simulink model "TRAS_closed_loop_"  (R2024b)
settings: Solver=FixedStepAuto  StartTime=0.0  StopTime=stop_time  FixedStep=sampling_time  RelTol=1e-3
values from neighbouring files (symbols this model uses):
  A = 0.0552    [momentsOfInertia.m]
  B = 0.0599    [momentsOfInertia.m]
  C = 0.0084    [momentsOfInertia.m]
  D = (mmr + mms + mm / 3) * lm^2 + (mtr + mts + mt / 3) * lt^2    (= 0.0224143186667)    [momentsOfInertia.m]
  E = mcb * lcb^2 + mb * lb^2 / 3    (= 0.0006225)    [momentsOfInertia.m]    (also in propeller_model.m = 12)
  F = mms * rms^2 + mts * rts^2    (= 0.002355075)    [momentsOfInertia.m]
  Fh_of_u2 = [zeros(1, len - length(Fh_of_u2)), Fh_of_u2] + [zeros(1, len - length(term)), term]    [thrustForcesDependencies.m]
  Fv_of_u1 = [zeros(1, len - length(Fv_of_u1)), Fv_of_u1] + [zeros(1, len - length(term)), term]    [thrustForcesDependencies.m]
  g = 9.81    [TRAS_closed_loop.m]    (also in TRAS_controller.m; TRAS_process.m)
  Jv = D + E + F    (= 0.0253918936667)    [momentsOfInertia.m]
  kd = 2 * zeta * wn + pole    (= 8.88888888889)    [TRAS_closed_loop.m]    (also in TRAS_controller.m = 4)
  kp = wn^2 + 2 * zeta * wn * pole    (= 15.890260631)    [TRAS_closed_loop.m]    (also in TRAS_controller.m = 4)
  L = (mmr + mms + mm / 4) * lm^2 + (mtr + mts + mt / 4) * lt^2 - mcb * lcb^2 - mb / 4 * lb^2    (= 0.021593306)    [momentsOfInertia.m]
  lm = 0.202    [momentsOfInertia.m]
  lt = 0.216    [momentsOfInertia.m]
  sampling_time = 1e-2    (= 0.01)    [TRAS_closed_loop.m]    (also in TRAS_controller.m; TRAS_process.m = 0.001; identification.m)
  x_grid = linspace(-4000, 4000, 1e4)    [TRAS_closed_loop.m]    (also in TRAS_controller.m = linspace(-1, 1, 1e5))
  y_grid_h = polyval(Fh, x_grid)    [TRAS_closed_loop.m]    (also in TRAS_controller.m = polyval(Fh_of_u2, x_grid))
  y_grid_v = polyval(Fv, x_grid)    [TRAS_closed_loop.m]    (also in TRAS_controller.m = polyval(Fv_of_u1, x_grid))
libraries: simulink x2, eeGeneralControl x2
settings Model: Creator=Codrin  LastModifiedBy=Codrin

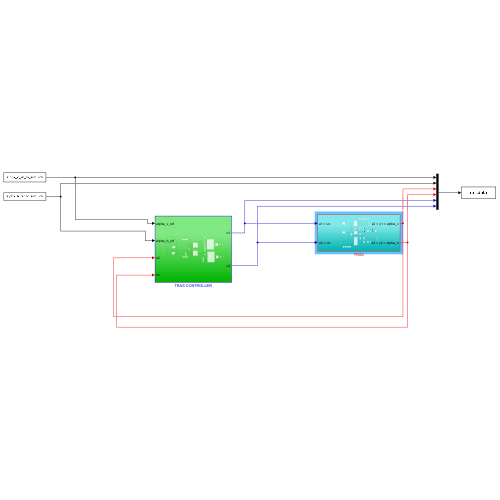
[thumbnail: Simulink's stored preview of the top-level diagram]
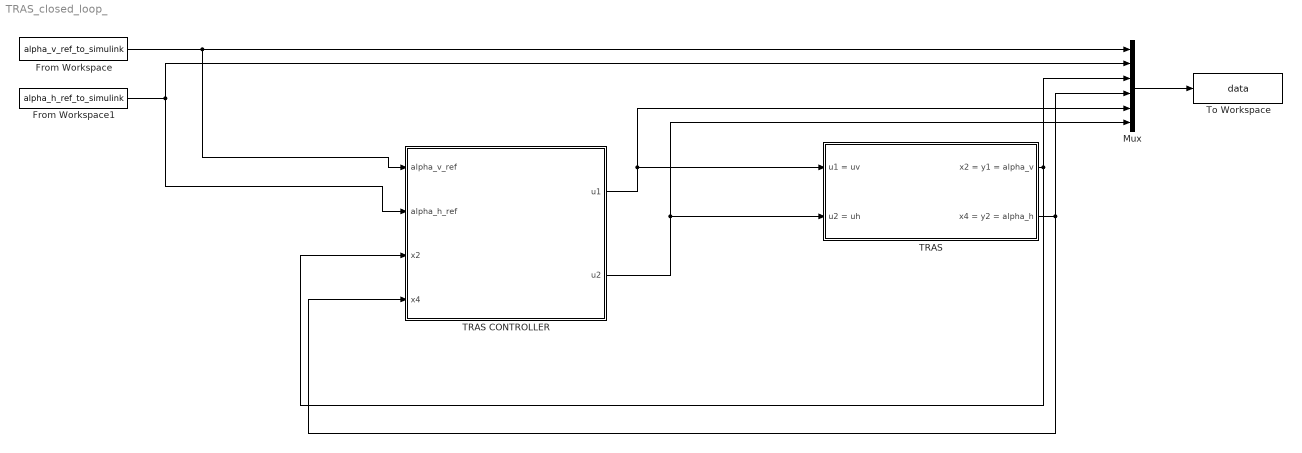
== system TRAS_closed_loop_ ==
  From Workspace : FromWorkspace  VariableName=alpha_v_ref_to_simulink
  From Workspace1 : FromWorkspace  VariableName=alpha_h_ref_to_simulink
  Mux : Mux  Inputs=6
  TRAS : Subsystem
  TRAS CONTROLLER : Subsystem
  To Workspace : ToWorkspace  VariableName=data  SaveFormat=Timeseries  SampleTime=-1
  wires:
  TRAS/2(x4 = y2 = alpha_h) -> TRAS CONTROLLER/4(x4), Mux/4
  Mux/1 -> To Workspace/1
  TRAS/1(x2 = y1 = alpha_v) -> TRAS CONTROLLER/3(x2), Mux/3
  TRAS CONTROLLER/1(u1) -> Mux/5, TRAS/1(u1 = uv)
  TRAS CONTROLLER/2(u2) -> Mux/6, TRAS/2(u2 = uh)
  From Workspace/1 -> TRAS CONTROLLER/1(alpha_v_ref), Mux/1
  From Workspace1/1 -> TRAS CONTROLLER/2(alpha_h_ref), Mux/2

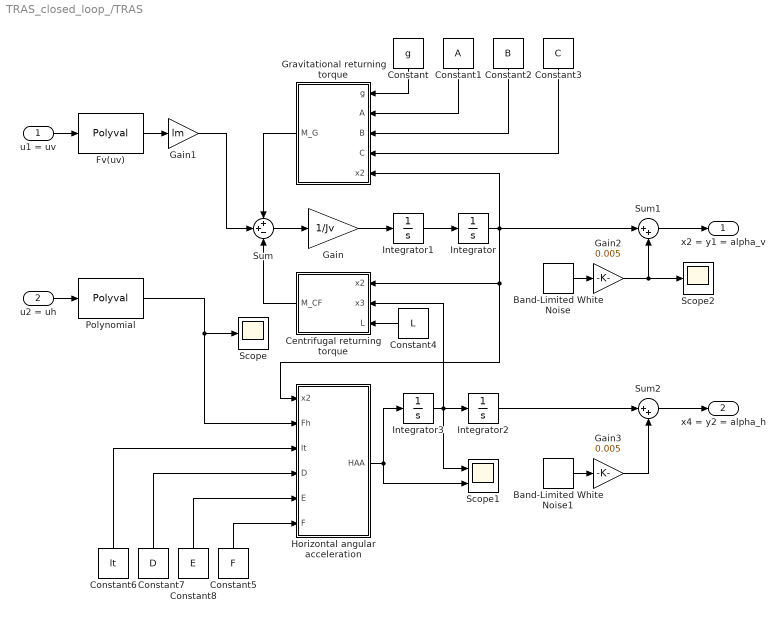
== system TRAS_closed_loop_/TRAS ==
  u1 = uv : Inport
  u2 = uh : Inport  Port=2
  Band-Limited White Noise : simulink/Sources/Band-Limited White Noise  Cov=[0.01]  Ts=sampling_time  seed=[23341]
  Band-Limited White Noise1 : simulink/Sources/Band-Limited White Noise  Cov=[0.01]  Ts=sampling_time  seed=[23341]
  Centrifugal returning torque : MATLAB Function  TreatAsAtomicUnit=on
  Constant : Constant  Value=g
  Constant1 : Constant  Value=A
  Constant2 : Constant  Value=B
  Constant3 : Constant  Value=C
  Constant4 : Constant  Value=L
  Constant5 : Constant  Value=F
  Constant6 : Constant  Value=lt
  Constant7 : Constant  Value=D
  Constant8 : Constant  Value=E
  Fv(uv) : Polyval  Coefs=Fv_of_u1
  Gain : Gain  Gain=1/Jv
  Gain1 : Gain  Gain=lm
  Gain2 : Gain  Gain=0.005
  Gain3 : Gain  Gain=0.005
  Gravitational returning torque : MATLAB Function  TreatAsAtomicUnit=on
  Horizontal angular acceleration : MATLAB Function  TreatAsAtomicUnit=on
  Integrator{,1..3} (4 alike) : Integrator
  Polynomial : Polyval  Coefs=Fh_of_u2
  Scope : Scope
  Scope1 : Scope  NumInputPorts=2
  Scope2 : Scope
  Sum : Sum  Inputs=++-
  Sum1 : Sum  Inputs=|++
  Sum2 : Sum  Inputs=|++
  x2 = y1 = alpha_v : Outport
  x4 = y2 = alpha_h : Outport  Port=2
  wires:
  u1 = uv/1 -> Fv(uv)/1
  Integrator/1 -> Sum1/1, Gravitational returning torque/5(x2), Horizontal angular acceleration/1(x2), Centrifugal returning torque/1(x2)
  Integrator1/1 -> Integrator/1
  Gain/1 -> Integrator1/1
  Sum/1 -> Gain/1
  Gravitational returning torque/1(M_G) -> Sum/1
  Fv(uv)/1 -> Gain1/1
  Gain1/1 -> Sum/2
  Centrifugal returning torque/1(M_CF) -> Sum/3
  Integrator3/1 -> Integrator2/1, Scope1/1, Centrifugal returning torque/2(x3)
  u2 = uh/1 -> Polynomial/1
  Constant/1 -> Gravitational returning torque/1(g)
  Constant1/1 -> Gravitational returning torque/2(A)
  Constant2/1 -> Gravitational returning torque/3(B)
  Constant3/1 -> Gravitational returning torque/4(C)
  Constant4/1 -> Centrifugal returning torque/3(L)
  Constant5/1 -> Horizontal angular acceleration/6(F)
  Constant8/1 -> Horizontal angular acceleration/5(E)
  Constant7/1 -> Horizontal angular acceleration/4(D)
  Constant6/1 -> Horizontal angular acceleration/3(lt)
  Polynomial/1 -> Horizontal angular acceleration/2(Fh), Scope/1
  Horizontal angular acceleration/1(HAA) -> Integrator3/1, Scope1/2
  Sum1/1 -> x2 = y1 = alpha_v/1
  Sum2/1 -> x4 = y2 = alpha_h/1
  Integrator2/1 -> Sum2/1
  Band-Limited White Noise1/1 -> Gain3/1
  Gain3/1 -> Sum2/2
  Band-Limited White Noise/1 -> Gain2/1
  Gain2/1 -> Scope2/1, Sum1/2

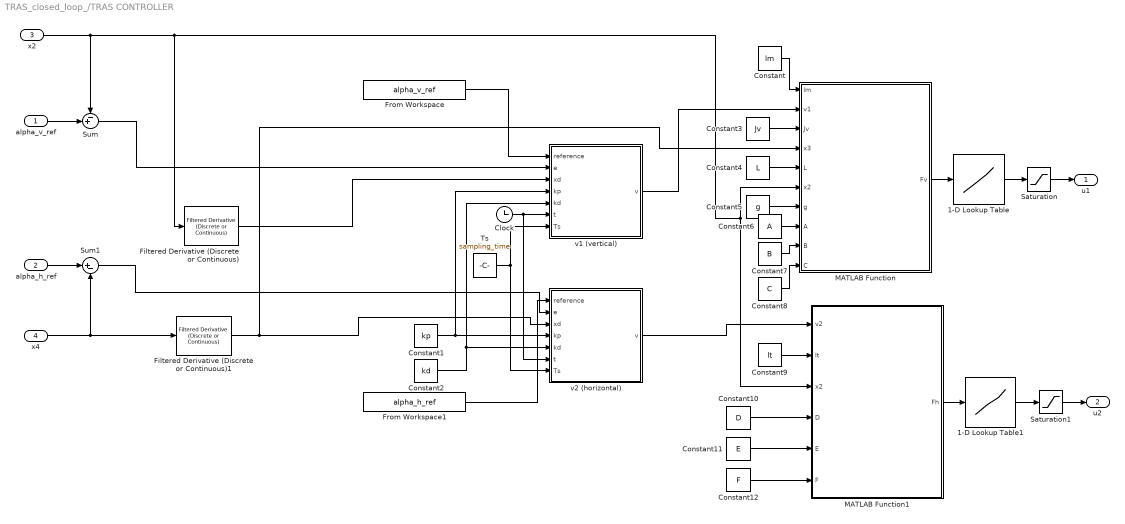
== system TRAS_closed_loop_/TRAS CONTROLLER ==
  alpha_v_ref : Inport
  alpha_h_ref : Inport  Port=2
  x2 : Inport  Port=3
  x4 : Inport  Port=4
  1-D Lookup Table : Lookup_n-D  NumberOfTableDimensions=1  BreakpointsForDimension1=y_grid_v  Table=x_grid  InterpMethod=Cubic spline  InternalRulePriority=Speed  RndMeth=Simplest
  1-D Lookup Table1 : Lookup_n-D  NumberOfTableDimensions=1  BreakpointsForDimension1=y_grid_h  Table=x_grid  InternalRulePriority=Speed  RndMeth=Simplest
  Clock : Clock
  Constant : Constant  Value=lm
  Constant1 : Constant  Value=kp
  Constant10 : Constant  Value=D
  Constant11 : Constant  Value=E
  Constant12 : Constant  Value=F
  Constant2 : Constant  Value=kd
  Constant3 : Constant  Value=Jv
  Constant4 : Constant  Value=L
  Constant5 : Constant  Value=g
  Constant6 : Constant  Value=A
  Constant7 : Constant  Value=B
  Constant8 : Constant  Value=C
  Constant9 : Constant  Value=lt
  Filtered Derivative (Discrete or Continuous) : eeGeneralControl/Filtered Derivative (Discrete or Continuous)  K=1  T=0.2  B=inf  A=-inf  minRatio=10  init_option=Inherited from block input  x0=0  Ts=-1
      settings: LibrarySourceBlock=|
      | ee_sl_lib/General Control/Filtered Derivative
      | (Discrete or Continuous)
  Filtered Derivative (Discrete or Continuous)1 : eeGeneralControl/Filtered Derivative (Discrete or Continuous)  K=1  T=0.2  B=inf  A=-inf  minRatio=10  init_option=Inherited from block input  x0=0  Ts=-1
      settings: LibrarySourceBlock=|
      | ee_sl_lib/General Control/Filtered Derivative
      | (Discrete or Continuous)
  From Workspace : FromWorkspace  VariableName=alpha_v_ref
  From Workspace1 : FromWorkspace  VariableName=alpha_h_ref
  MATLAB Function : MATLAB Function  TreatAsAtomicUnit=on
  MATLAB Function1 : MATLAB Function  TreatAsAtomicUnit=on
  Saturation : Saturate  UpperLimit=0.98  LowerLimit=-0.98
  Saturation1 : Saturate  UpperLimit=0.98  LowerLimit=-0.98
  Sum : Sum  Inputs=-+|
  Sum1 : Sum  Inputs=|+-
  Ts : Constant  Value=sampling_time
  v1 (vertical) : MATLAB Function  TreatAsAtomicUnit=on
  v2 (horizontal) : MATLAB Function  TreatAsAtomicUnit=on
  u1 : Outport
  u2 : Outport  Port=2
  wires:
  Clock/1 -> v2 (horizontal)/6(t), v1 (vertical)/6(t)
  Ts/1 -> v2 (horizontal)/7(Ts), v1 (vertical)/7(Ts)
  Constant1/1 -> v1 (vertical)/4(kp), v2 (horizontal)/4(kp)
  Constant2/1 -> v1 (vertical)/5(kd), v2 (horizontal)/5(kd)
  From Workspace1/1 -> v2 (horizontal)/1(reference)
  From Workspace/1 -> v1 (vertical)/1(reference)
  Filtered Derivative (Discrete or Continuous)/1 -> v1 (vertical)/3(xd)
  Filtered Derivative (Discrete or Continuous)1/1 -> v2 (horizontal)/3(xd), MATLAB Function/4(x3)
  Constant/1 -> MATLAB Function/1(lm)
  v1 (vertical)/1(v) -> MATLAB Function/2(v1)
  Constant3/1 -> MATLAB Function/3(Jv)
  Constant4/1 -> MATLAB Function/5(L)
  x2/1 -> Sum/1, Filtered Derivative (Discrete or Continuous)/1, MATLAB Function1/3(x2), MATLAB Function/6(x2)
  Constant5/1 -> MATLAB Function/7(g)
  Constant6/1 -> MATLAB Function/8(A)
  Constant7/1 -> MATLAB Function/9(B)
  Constant8/1 -> MATLAB Function/10(C)
  v2 (horizontal)/1(v) -> MATLAB Function1/1(v2)
  Constant9/1 -> MATLAB Function1/2(lt)
  Constant10/1 -> MATLAB Function1/4(D)
  Constant11/1 -> MATLAB Function1/5(E)
  Constant12/1 -> MATLAB Function1/6(F)
  MATLAB Function/1(Fv) -> 1-D Lookup Table/1
  MATLAB Function1/1(Fh) -> 1-D Lookup Table1/1
  1-D Lookup Table/1 -> Saturation/1
  Saturation/1 -> u1/1
  Saturation1/1 -> u2/1
  1-D Lookup Table1/1 -> Saturation1/1
  x4/1 -> Sum1/2, Filtered Derivative (Discrete or Continuous)1/1
  Sum/1 -> v1 (vertical)/2(e)
  alpha_v_ref/1 -> Sum/2
  alpha_h_ref/1 -> Sum1/1
  Sum1/1 -> v2 (horizontal)/2(e)

== matlab function TRAS_closed_loop_/TRAS/Centrifugal returning torque ==
  data: x2 input; M_CF output; x3 input; L input
function M_CF = M_CF(x2, x3, L)

M_CF = x3^2 / 2 * L * sin(2 * x2);

== matlab function TRAS_closed_loop_/TRAS/Gravitational returning torque ==
  data: g input; A input; B input; C input; x2 input; M_G output
function M_G = M_G(g, A, B, C, x2)

M_G = g * ((A - B) * cos(x2) - C * sin(x2));

== matlab function TRAS_closed_loop_/TRAS/Horizontal angular acceleration ==
  data: x2 input; Fh input; HAA output; lt input; D input; E input; F input
function HAA = HAA(x2, Fh, lt, D, E, F)

HAA = lt * Fh * cos(x2) / (D * cos(x2)^2 + E * sin(x2)^2 + F);

== matlab function TRAS_closed_loop_/TRAS CONTROLLER/v1 (vertical) ==
  data: reference input; v output; e input; xd input; kp input; kd input; t input; Ts input
function v = v_computation(reference, e, xd, kp, kd, t, Ts)

%reference = reference signal
%e = error
%xd = state that intervenes in the first derivative of the error

step = round(t / Ts) + 1;

reference = [reference(1); reference; reference(end); reference(end)];
referenced = (reference(step + 2) - reference(step)) / (2 * Ts);
referencedd = (reference(step + 2) - 2 * reference(step + 1) + reference(step)) / (Ts ^ 2);

v = referencedd + kd * (referenced - xd) + kp * e;

== matlab function TRAS_closed_loop_/TRAS CONTROLLER/v2 (horizontal) ==
  data: reference input; v output; e input; xd input; kp input; kd input; t input; Ts input
function v = v_computation(reference, e, xd, kp, kd, t, Ts)

%reference = reference signal
%e = error
%xd = state that intervenes in the first derivative of the error

step = round(t / Ts) + 1;

reference = [reference(1); reference; reference(end); reference(end)];
referenced = (reference(step + 2) - reference(step)) / (2 * Ts);
referencedd = (reference(step + 2) - 2 * reference(step + 1) + reference(step)) / (Ts ^ 2);

v = referencedd + kd * (referenced - xd) + kp * e;

== matlab function TRAS_closed_loop_/TRAS CONTROLLER/MATLAB Function ==
  data: lm input; Fv output; v1 input; Jv input; x3 input; L input; x2 input; g input; A input; B input; C input
function Fv = verticalForceComputation(lm, v1, Jv, x3, L, x2, g, A, B, C)

Fv = 1 / lm * (v1 * Jv + x3^2 / 2 * L * sin(2 * x2) - g * ((A-B)*cos(x2) - C*sin(x2)));

== matlab function TRAS_closed_loop_/TRAS CONTROLLER/MATLAB Function1 ==
  data: v2 input; Fh output; lt input; x2 input; D input; E input; F input
function Fh = horizontalForceComputation(v2, lt, x2, D, E, F)

Fh = v2 / (lt * cos(x2)) * (D * cos(x2)^2 + E * sin(x2)^2 + F);
